simulink model "aaa1"  (R2021b)
settings: Solver=VariableStepAuto  StartTime=0.0  StopTime=50  RelTol=1e-3
libraries: simulink x3
settings Model: Creator=郭义月  LastModifiedBy=郭义月

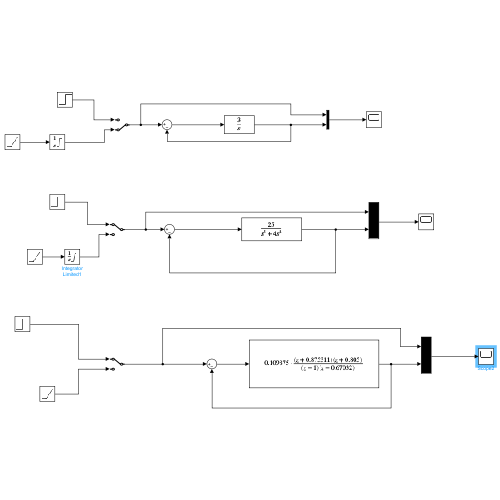
[thumbnail: Simulink's stored preview of the top-level diagram]
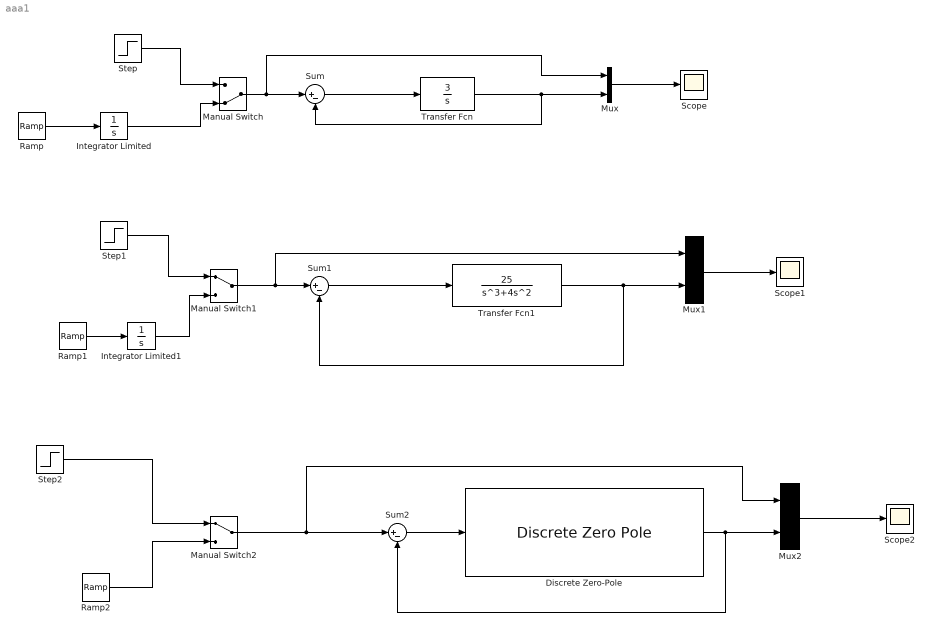
== system aaa1 ==
  Discrete Zero-Pole : DiscreteZeroPole  Zeros=[-0.875311 -0.805]  Poles=[1 0.67032]  Gain=0.109875  SampleTime=-1
  Integrator Limited : Integrator  LimitOutput=on  UpperSaturationLimit=1000  LowerSaturationLimit=0
  Integrator Limited1 : Integrator  LimitOutput=on  UpperSaturationLimit=1000  LowerSaturationLimit=0
  Manual Switch : ManualSwitch  CurrentSetting=0
  Manual Switch1 : ManualSwitch
  Manual Switch2 : ManualSwitch
  Mux : Mux  Inputs=2
  Mux1 : Mux  Inputs=2
  Mux2 : Mux  Inputs=2
  Ramp : simulink/Sources/Ramp  slope=1  start=0  InitialOutput=0
  Ramp1 : simulink/Sources/Ramp  slope=1  start=0  InitialOutput=0
  Ramp2 : simulink/Sources/Ramp  slope=1  start=0  InitialOutput=0
  Scope : Scope
  Scope1 : Scope
  Scope2 : Scope
  Step : Step  SampleTime=0
  Step1 : Step  SampleTime=0
  Step2 : Step  SampleTime=0
  Sum : Sum  Inputs=|+-
  Sum1 : Sum  Inputs=|+-
  Sum2 : Sum  Inputs=|+-
  Transfer Fcn : TransferFcn  Numerator=[3]  Denominator=[1 0]
  Transfer Fcn1 : TransferFcn  Numerator=[25]  Denominator=[1 4 0 0]
  wires:
  Step/1 -> Manual Switch/1
  Ramp/1 -> Integrator Limited/1
  Sum/1 -> Transfer Fcn/1
  Transfer Fcn/1 -> Mux/2, Sum/2
  Mux/1 -> Scope/1
  Manual Switch/1 -> Mux/1, Sum/1
  Step1/1 -> Manual Switch1/1
  Ramp1/1 -> Integrator Limited1/1
  Manual Switch1/1 -> Mux1/1, Sum1/1
  Sum1/1 -> Transfer Fcn1/1
  Transfer Fcn1/1 -> Mux1/2, Sum1/2
  Mux1/1 -> Scope1/1
  Ramp2/1 -> Manual Switch2/2
  Sum2/1 -> Discrete Zero-Pole/1
  Manual Switch2/1 -> Mux2/1, Sum2/1
  Discrete Zero-Pole/1 -> Mux2/2, Sum2/2
  Mux2/1 -> Scope2/1
  Integrator Limited/1 -> Manual Switch/2
  Integrator Limited1/1 -> Manual Switch1/2
  Step2/1 -> Manual Switch2/1
